simulink model "dc_motor_control_system"  (R2019a)
settings: Solver=VariableStepAuto  StartTime=0.0  StopTime=10.0  RelTol=1e-3
undefined symbols (not defined in the file or in its folder): TS
settings Model: Creator=takis  LastModifiedBy=takis

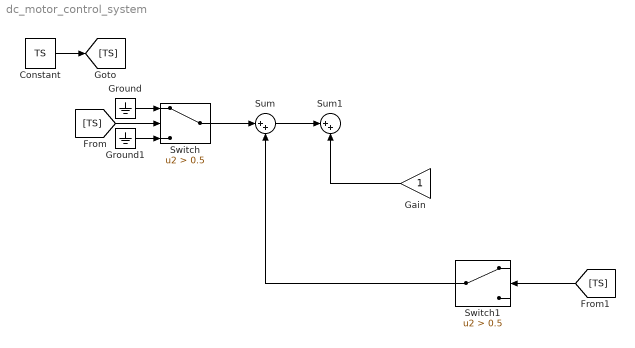
== system dc_motor_control_system ==
  Constant : Constant  Value=TS
  Gain : Gain
  Ground : Ground
  Ground1 : Ground
  Sum : Sum  Inputs=|++
  Sum1 : Sum  Inputs=|++
  Switch : Switch  Criteria=u2 > Threshold  Threshold=0.5
  Switch1 : Switch  Criteria=u2 > Threshold  Threshold=0.5
  wires:
  Gain/1 -> Sum1/2
  Sum/1 -> Sum1/1
  Switch/1 -> Sum/1
  [TS] -> Switch/2
  [TS] -> Switch1/2
  Constant/1 -> [TS]
  Ground/1 -> Switch/1
  Ground1/1 -> Switch/3
  Switch1/1 -> Sum/2
